simulink model "Gradient_Descent_Sleep"  (R2015a)
settings: Solver=ode3  StartTime=0.0  StopTime=320  FixedStep=0.01  MaxStep=0.01  RelTol=1e-3
values from neighbouring files (symbols this model uses):
  H0 = interp1q(Periodic_Solution(:,1),Periodic_Solution(:,4),Initial_Time)    [Gradient_Descent_Controllable_Sleeping.m]    (also in Model_Simplification.m = interp1q(Periodic_Solution(:,1),Periodic_Solution(:,4),time_)
  I_update = I    [Gradient_Descent_Controllable_Sleeping.m]    (also in Model_Simplification.m = u;I_update(:,2)=I_update(:,2)*Imax/umax)
  n0 = interp1q(Periodic_Solution(:,1),Periodic_Solution(:,7),Initial_Time)    [Gradient_Descent_Controllable_Sleeping.m]    (also in Model_Simplification.m = interp1q(Periodic_Solution(:,1),Periodic_Solution(:,7),time_)
  Periodic_Solution = Periodic_Solution(Initial_Time*100+time_shift(nn)*100+1:end,:)    [Gradient_Descent_Controllable_Sleeping.m]    (also in Model_Simplification.m = Periodic_Solution(Initial_Time*100+1:end,:); plot_sleepiness.m = Periodic_Solution(Initial_Time*100+1:end,:))
  Sleep0 = 0    [Gradient_Descent_Controllable_Sleeping.m]    (also in Model_Simplification.m)
  Sleep_update = Sleep    [Gradient_Descent_Controllable_Sleeping.m]    (also in Model_Simplification.m = sleep)
  tol = 0.01    [Gradient_Descent_Controllable_Sleeping.m]    (also in Model_Simplification.m; plot_sleepiness.m)
  x0 = interp1q(Periodic_Solution(:,1),Periodic_Solution(:,2),Initial_Time)    [Gradient_Descent_Controllable_Sleeping.m]    (also in Model_Simplification.m = interp1q(Periodic_Solution(:,1),Periodic_Solution(:,2),time_)
  xc0 = interp1q(Periodic_Solution(:,1),Periodic_Solution(:,3),Initial_Time)    [Gradient_Descent_Controllable_Sleeping.m]    (also in Model_Simplification.m = interp1q(Periodic_Solution(:,1),Periodic_Solution(:,3),time_)
settings Model: Creator=wangf7  LastModifiedBy=Jiawei Yin
settings OptimizationCC: ExpressionDepthLimit=2147483647
settings DebuggingCC: AlgebraicLoopMsg=none  ArtificialAlgebraicLoopMsg=none  UnderspecifiedInitializationDetection=Classic  MergeDetectMultiDrivingBlocksExec=none  SolverPrmCheckMsg=warning  StateNameClashWarn=warning

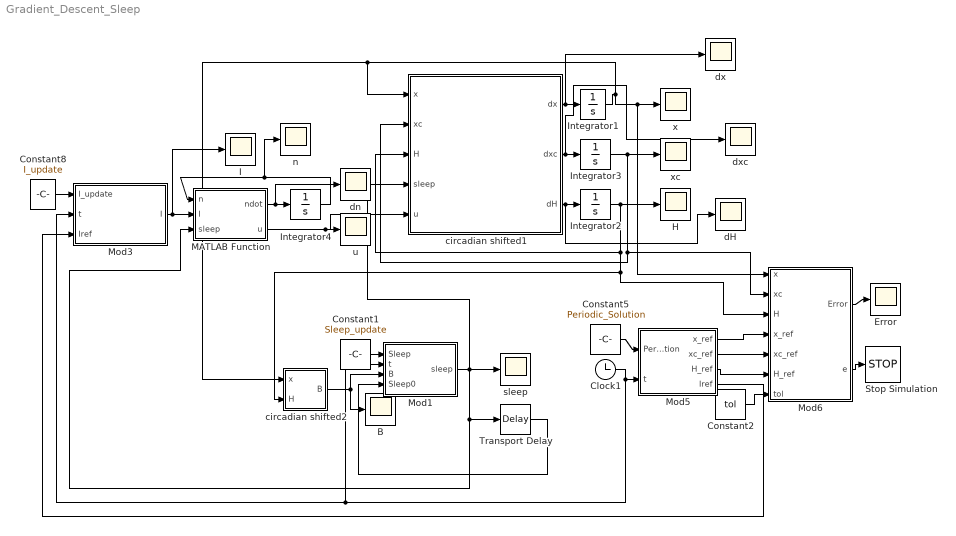
== system Gradient_Descent_Sleep ==
  B : Scope
      settings: TimeRange=auto  MaxDataPoints=5000000000  SaveName=B_plus  YMin=0.1808  YMax=0.82676  SampleTime=-1  DataFormat=Array
  Clock1 : Clock
  Constant1 : Constant  Value=Sleep_update
  Constant2 : Constant  Value=tol
  Constant5 : Constant  Value=Periodic_Solution
  Constant8 : Constant  Value=I_update
  Error : Scope
      settings: TimeRange=auto  MaxDataPoints=5000000000  SaveName=Error  YMin=-0.08503  YMax=0.86612  SampleTime=-1  DataFormat=Array
  H : Scope
      settings: TimeRange=auto  MaxDataPoints=5000000000  SaveName=H  YMin=0.55428  YMax=0.67222  SampleTime=-1  DataFormat=Array
  I : Scope
      settings: TimeRange=auto  MaxDataPoints=5000  SaveName=I  YMin=-1250.00000  YMax=11250.00000  SampleTime=-1  DataFormat=Array
  Integrator1 : Integrator  InitialCondition=x0
  Integrator2 : Integrator  InitialCondition=H0
  Integrator3 : Integrator  InitialCondition=xc0
  Integrator4 : Integrator  InitialCondition=n0
  MATLAB Function : MATLAB Function  TreatAsAtomicUnit=on
      settings: PermitHierarchicalResolution=ParametersOnly
  Mod1 : MATLAB Function  TreatAsAtomicUnit=on
      settings: PermitHierarchicalResolution=ParametersOnly
  Mod3 : MATLAB Function  TreatAsAtomicUnit=on
      settings: PermitHierarchicalResolution=ParametersOnly
  Mod5 : MATLAB Function  TreatAsAtomicUnit=on
      settings: PermitHierarchicalResolution=ParametersOnly
  Mod6 : MATLAB Function  TreatAsAtomicUnit=on
      settings: PermitHierarchicalResolution=ParametersOnly
  Stop Simulation : Stop
  Transport Delay : TransportDelay  DelayTime=.01  InitialOutput=Sleep0
  circadian shifted1 : MATLAB Function  TreatAsAtomicUnit=on
      settings: PermitHierarchicalResolution=ParametersOnly
  circadian shifted2 : MATLAB Function  TreatAsAtomicUnit=on
      settings: PermitHierarchicalResolution=ParametersOnly
  dH : Scope
      settings: TimeRange=auto  MaxDataPoints=5000000000  SaveName=dH  YMin=-0.17252  YMax=0.04653  SampleTime=-1  DataFormat=Array
  dn : Scope
      settings: TimeRange=auto  MaxDataPoints=5000000000  SaveName=dn  YMin=-0.73175  YMax=2.66539  SampleTime=-1  DataFormat=Array
  dx : Scope
      settings: TimeRange=auto  MaxDataPoints=5000000000  SaveName=dx  YMin=-0.39269  YMax=0.10123  SampleTime=-1  DataFormat=Array
  dxc : Scope
      settings: TimeRange=auto  MaxDataPoints=5000000000  SaveName=dxc  YMin=-0.78535  YMax=7.06815  SampleTime=-1  DataFormat=Array
  n : Scope
      settings: TimeRange=auto  MaxDataPoints=5000000000  SaveName=n  YMin=-0.08228  YMax=0.97853  SampleTime=-1  DataFormat=Array
  sleep : Scope
      settings: TimeRange=auto  MaxDataPoints=5000000000  SaveName=Sleep  YMin=-0.125  YMax=1.125  SampleTime=-1  DataFormat=Array
  u : Scope
      settings: TimeRange=auto  MaxDataPoints=5000000000  SaveName=u  YMin=0.55428  YMax=0.67222  SampleTime=-1  DataFormat=Array
  x : Scope
      settings: TimeRange=auto  MaxDataPoints=5000000000  SaveName=x  YMin=-0.78535  YMax=7.06815  SampleTime=-1  DataFormat=Array
  xc : Scope
      settings: TimeRange=auto  MaxDataPoints=5000000000  SaveName=xc  YMin=0.55428  YMax=0.67222  SampleTime=-1  DataFormat=Array
  wires:
  circadian shifted1/1(dx) -> dx/1, Integrator1/1
  circadian shifted1/2(dxc) -> dxc/1, Integrator3/1
  Integrator1/1 -> x/1, Mod6/1(x), circadian shifted1/1(x), circadian shifted2/1(x)
  Integrator3/1 -> circadian shifted1/2(xc), Mod6/2(xc), xc/1
  Constant5/1 -> Mod5/1(Periodic_Solution)
  Mod6/2(e) -> Stop Simulation/1
  Mod6/1(Error) -> Error/1
  Mod5/3(H_ref) -> Mod6/6(H_ref)
  Constant2/1 -> Mod6/7(tol)
  Constant1/1 -> Mod1/1(Sleep)
  Clock1/1 -> Mod1/2(t), Mod3/2(t), Mod5/2(t)
  Mod1/1(sleep) -> circadian shifted1/4(sleep), MATLAB Function/3(sleep), Transport Delay/1, sleep/1
  circadian shifted2/1(B) -> Mod1/3(B), B/1
  Transport Delay/1 -> Mod1/4(Sleep0)
  circadian shifted1/3(dH) -> Integrator2/1, dH/1
  Integrator2/1 -> Mod6/3(H), circadian shifted2/2(H), circadian shifted1/3(H), H/1
  Mod5/1(x_ref) -> Mod6/4(x_ref)
  Mod5/2(xc_ref) -> Mod6/5(xc_ref)
  Constant8/1 -> Mod3/1(I_update)
  MATLAB Function/2(u) -> circadian shifted1/5(u), u/1
  MATLAB Function/1(ndot) -> dn/1, Integrator4/1
  Integrator4/1 -> n/1, MATLAB Function/1(n)
  Mod3/1(I) -> I/1, MATLAB Function/2(I)
  Mod5/4(Iref) -> Mod3/3(Iref)

== matlab function Gradient_Descent_Sleep/circadian shifted1 ==
  data: x input; xc input; H input; sleep input; u input; dx output; dxc output; dH output
function [ dx,dxc,dH] = fcn(x,xc,H,sleep,u)
%#eml

tr=18.2;
td=4.2;

q = 1/3;
taux = 24.2;
k = 0.55;
mu=0.13;

B = u*(1-sleep)*(1-0.4*x)*(1-0.4*xc);

dx = (pi/12)*(xc + B  + mu*(1/3*x + 4/3*x^3 - 256/105*x^7));
dxc = (pi/12)*(q*B *xc - (24/(taux*0.99729))^2*x - k*B*x);
dH = (1-sleep)*(1-H)/tr-(H*sleep)/td;

== matlab function Gradient_Descent_Sleep/Mod1 ==
  data: Sleep input; sleep output; t input; B input; Sleep0 input
function sleep = fcn(Sleep,t,B,Sleep0)
%#codegen
if t<=Sleep(end,1)
    sleep=interp1q(Sleep(:,1),Sleep(:,2),t);
    if sleep==0 && round(Sleep0)==1
        if B>0.27
            sleep=1;
        end
    elseif sleep==1 && round(Sleep0)==0
        if B<0.67
            sleep=0;
        end
    end
    if B>0.77
        sleep=1;
    elseif B<0.17
        sleep=0;
    end
else
    sleep=round(Sleep0);
    if B>0.67
        sleep=1;
    elseif B<0.17
        sleep=0;
    end
end

== matlab function Gradient_Descent_Sleep/circadian shifted2 ==
  data: x input; H input; B output
function B = fcn(x,H)
%#eml
B=H-0.1333*x;

== matlab function Gradient_Descent_Sleep/MATLAB Function ==
  data: n input; I input; ndot output; u output; sleep input
function [ndot,u] = fcn(n,I,sleep)
G=33.75;
alpha0=0.05;
beta=0.0075;
I0=9500;
alpha=alpha0*(I/I0)^0.5;
u=G*alpha*(1-n)*(1-sleep);
ndot=60*[alpha*(1-n)*(1-sleep)-beta*n];

== matlab function Gradient_Descent_Sleep/Mod5 ==
  data: Periodic_Solution input; x_ref output; xc_ref output; t input; H_ref output; Iref output
function [x_ref,xc_ref,H_ref,Iref] = fcn(Periodic_Solution,t)
%#codegen
x_ref=interp1q(Periodic_Solution(:,1),Periodic_Solution(:,2),t);
xc_ref=interp1q(Periodic_Solution(:,1),Periodic_Solution(:,3),t);
H_ref=interp1q(Periodic_Solution(:,1),Periodic_Solution(:,4),t);
% Sleep_ref=interp1q(Periodic_Solution(:,1),Periodic_Solution(:,6),t);
Iref=interp1q(Periodic_Solution(:,1),Periodic_Solution(:,5),t);

== matlab function Gradient_Descent_Sleep/Mod6 ==
  data: Error output; x input; xc input; H input; x_ref input; xc_ref input; H_ref input; e output; tol input
function [Error,e] = fcn(x,xc,H,x_ref,xc_ref,H_ref,tol)
%#codegen
Error=(H-H_ref)^2+(x-x_ref)^2+(xc-xc_ref)^2;
e=Error<tol;

== matlab function Gradient_Descent_Sleep/Mod3 ==
  data: I_update input; I output; t input; Iref input
function I  = fcn(I_update,t,Iref)
%#codegen
if t<=I_update(end,1)
    I=interp1q(I_update(:,1),I_update(:,2),t);
else
    I=Iref;
end
